simulink model "mtpa_reference_wrapper"  (R2026a)
settings: Solver=FixedStepDiscrete  FixedStep=5e-5
libraries: mcbcontrolslib x1
settings Model: Creator=hzldx  LastModifiedBy=hzldx
settings RTWCC: SystemTargetFile=ert.tlc  GenCodeOnly=on  GenerateMakefile=off  Description=Embedded Coder

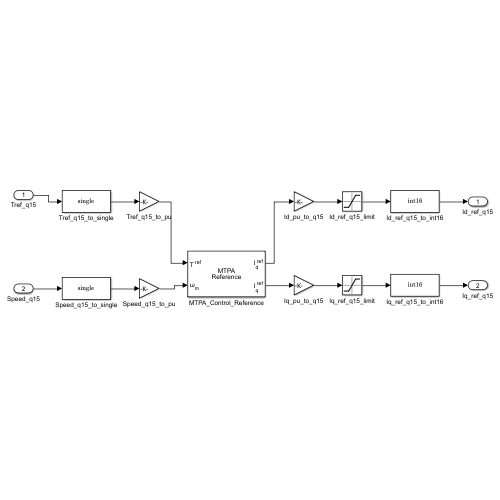
[thumbnail: Simulink's stored preview of the top-level diagram]
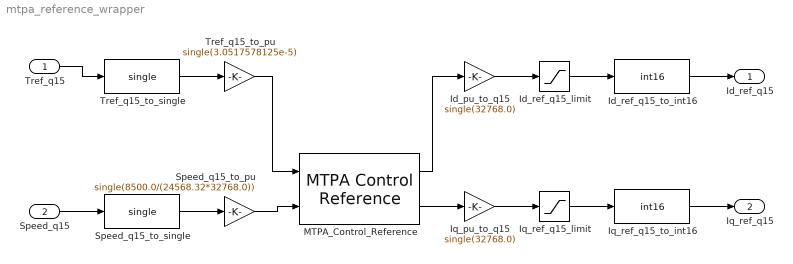
== system mtpa_reference_wrapper ==
  Tref_q15 : Inport  OutDataTypeStr=int16
  Speed_q15 : Inport  Port=2  OutDataTypeStr=int16
  Id_pu_to_q15 : Gain  Gain=single(32768.0)  OutDataTypeStr=single
  Id_ref_q15_limit : Saturate  UpperLimit=32767.0  LowerLimit=-32768.0
  Id_ref_q15_to_int16 : DataTypeConversion  OutDataTypeStr=int16
  Iq_pu_to_q15 : Gain  Gain=single(32768.0)  OutDataTypeStr=single
  Iq_ref_q15_limit : Saturate  UpperLimit=32767.0  LowerLimit=-32768.0
  Iq_ref_q15_to_int16 : DataTypeConversion  OutDataTypeStr=int16
  MTPA_Control_Reference : mcbcontrolslib/MTPA Control Reference  VariantSelect=Interior PMSM  polePairs=4  Rs=0.55  Ld=0.0012  Lq=0.0023  FluxPM=0.032390572606  ilimit=50  Vdc_input_select=Specify via dialog  V_dc=1000  Units=Per-Unit (PU)  N_base=24568.32  I_base=50  T_base=9.7172  V_base=1000/sqrt(3)  N_base_disp=3182  MTPAiterator=on  iterCount=10
      settings: LibrarySourceBlock=mcblib/Controls/Control Reference/MTPA Control Reference
  Speed_q15_to_pu : Gain  Gain=single(8500.0/(24568.32*32768.0))  OutDataTypeStr=single
  Speed_q15_to_single : DataTypeConversion  OutDataTypeStr=single  SaturateOnIntegerOverflow=off  RndMeth=Floor
  Tref_q15_to_pu : Gain  Gain=single(3.0517578125e-5)  OutDataTypeStr=single
  Tref_q15_to_single : DataTypeConversion  OutDataTypeStr=single  SaturateOnIntegerOverflow=off  RndMeth=Floor
  Id_ref_q15 : Outport  OutDataTypeStr=int16
  Iq_ref_q15 : Outport  Port=2  OutDataTypeStr=int16
  wires:
  Tref_q15/1 -> Tref_q15_to_single/1
  Tref_q15_to_single/1 -> Tref_q15_to_pu/1
  Tref_q15_to_pu/1 -> MTPA_Control_Reference/1
  Speed_q15/1 -> Speed_q15_to_single/1
  Speed_q15_to_single/1 -> Speed_q15_to_pu/1
  Speed_q15_to_pu/1 -> MTPA_Control_Reference/2
  MTPA_Control_Reference/1 -> Id_pu_to_q15/1
  Id_pu_to_q15/1 -> Id_ref_q15_limit/1
  Id_ref_q15_limit/1 -> Id_ref_q15_to_int16/1
  Id_ref_q15_to_int16/1 -> Id_ref_q15/1
  MTPA_Control_Reference/2 -> Iq_pu_to_q15/1
  Iq_pu_to_q15/1 -> Iq_ref_q15_limit/1
  Iq_ref_q15_limit/1 -> Iq_ref_q15_to_int16/1
  Iq_ref_q15_to_int16/1 -> Iq_ref_q15/1
